simulink model "business"  (Simulink 8.0)
settings: Solver=ode3  StartTime=0.0  StopTime=inf  FixedStep=Ts  RelTol=1e-3
undefined symbols (not defined in the file): effectPerUnit, employees, KiEmployeeController, KpEmployeeController, materialcost, price, productionCost, salary, Ts
settings Model: Creator=ägarenn  LastModifiedBy=ägarenn
settings OptimizationCC: InlineParams=on
settings DebuggingCC: SolverPrmCheckMsg=none

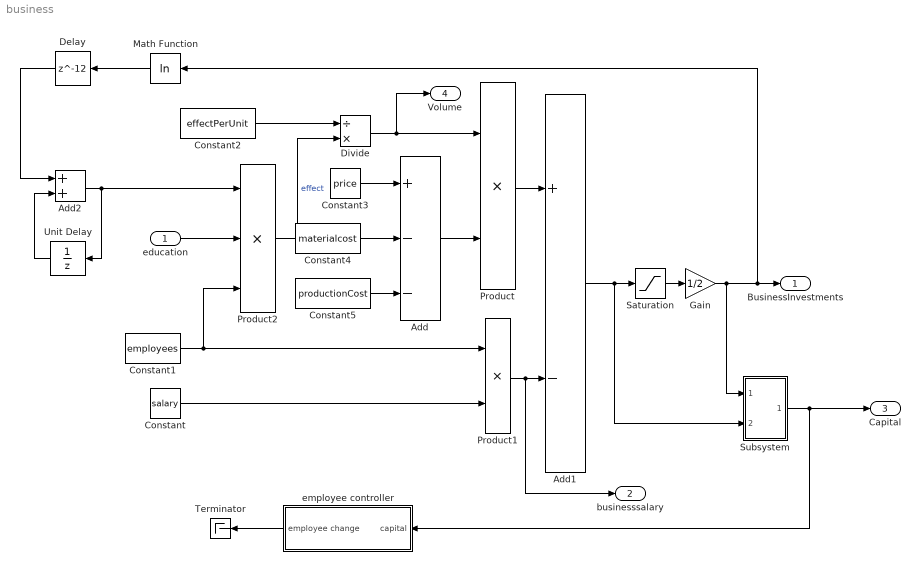
== system business ==
  education : Inport
  Add : Sum  Inputs=+--
  Add1 : Sum  Inputs=+-
  Add2 : Sum
  Constant : Constant  Value=salary
  Constant1 : Constant  Value=employees
  Constant2 : Constant  Value=effectPerUnit
  Constant3 : Constant  Value=price
  Constant4 : Constant  Value=materialcost
  Constant5 : Constant  Value=productionCost
  Delay : Delay  DelayLength=12
  Divide : Product  Inputs=/*
  Gain : Gain  Gain=1/2
  Math Function : Math  Operator=log  SaturateOnIntegerOverflow=on
  Product : Product  RndMeth=Zero
  Product1 : Product  RndMeth=Zero
  Product2 : Product  Inputs=3  RndMeth=Zero
  Saturation : Saturate  UpperLimit=inf  LowerLimit=2
  Subsystem : Subsystem
  Terminator : Terminator
  Unit Delay : UnitDelay  InitialCondition=1  SampleTime=-1
  employee controller : Subsystem
  BusinessInvestments : Outport
  businesssalary : Outport  Port=2
  Capital : Outport  Port=3
  Volume : Outport  Port=4
  wires:
  Constant1/1 -> Product2/3, Product1/1
  Constant/1 -> Product1/2
  Constant5/1 -> Add/3
  Constant3/1 -> Add/1
  Constant4/1 -> Add/2
  Add/1 -> Product/2
  Product/1 -> Add1/1
  Product1/1 -> businesssalary/1, Add1/2
  Saturation/1 -> Gain/1
  education/1 -> Product2/2
  Add2/1 -> Product2/1, Unit Delay/1
  Divide/1 -> Volume/1, Product/1
  Unit Delay/1 -> Add2/2
  Math Function/1 -> Delay/1
  Product2/1 -> Divide/2  "effect"
  Constant2/1 -> Divide/1
  Delay/1 -> Add2/1
  Add1/1 -> Subsystem/2(Result), Saturation/1
  Gain/1 -> Subsystem/1(Result/2), Math Function/1, BusinessInvestments/1
  Subsystem/1(Capital) -> employee controller/1(capital), Capital/1
  employee controller/1(employee change) -> Terminator/1

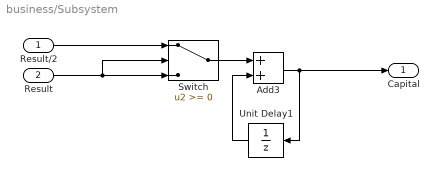
== system business/Subsystem ==
  Result/2 : Inport
  Result : Inport  Port=2
  Add3 : Sum
  Switch : Switch
  Unit Delay1 : UnitDelay  InitialCondition=10^10  SampleTime=-1
  Capital : Outport
  wires:
  Result/1 -> Switch/2, Switch/3
  Switch/1 -> Add3/1
  Add3/1 -> Capital/1, Unit Delay1/1
  Unit Delay1/1 -> Add3/2
  Result/2/1 -> Switch/1

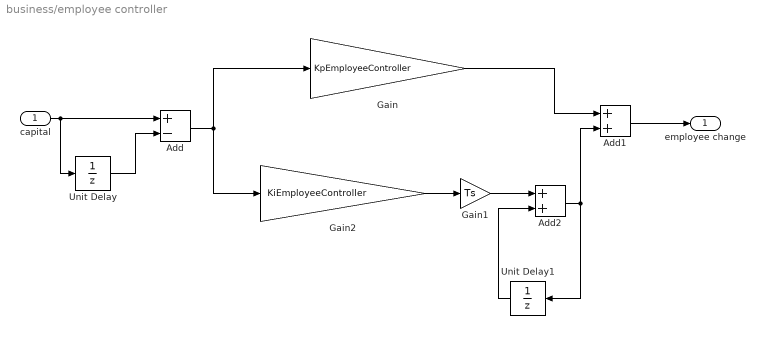
== system business/employee controller ==
  capital : Inport
  Add : Sum  Inputs=+-
  Add1 : Sum
  Add2 : Sum
  Gain : Gain  Gain=KpEmployeeController
  Gain1 : Gain  Gain=Ts
  Gain2 : Gain  Gain=KiEmployeeController
  Unit Delay : UnitDelay  SampleTime=-1
  Unit Delay1 : UnitDelay  SampleTime=-1
  employee change : Outport
  wires:
  capital/1 -> Add/1, Unit Delay/1
  Unit Delay/1 -> Add/2
  Add1/1 -> employee change/1
  Add/1 -> Gain2/1, Gain/1
  Gain/1 -> Add1/1
  Gain2/1 -> Gain1/1
  Add2/1 -> Unit Delay1/1, Add1/2
  Gain1/1 -> Add2/1
  Unit Delay1/1 -> Add2/2
